simulink model "project3_bonus_2016b"  (R2016b)
settings: Solver=ode23tb  StartTime=0.0  StopTime=inf  MaxStep=1  MinStep=1e-20  RelTol=1e-3
values from neighbouring files (symbols this model uses):
  C1 = 3.5e4    (= 35000)    [init.m]
  Np = 6    [init.m]
  Ns = 100    [init.m]
  Q_cell = Capacity*3600    (= 111600)    [init.m]
  R0 = 0.009    [init.m]
  R1 = 0.0015    [init.m]
  SOC_min = 0.2    [init.m]
undefined symbols (not defined in the file or in its folder): P_trac
libraries: simulink x1
settings Model: Creator=wasynczu  LastModifiedBy=wasynczu
settings SFSimCC: SimUseLocalCustomCode=on
settings RTWCC: RTWUseLocalCustomCode=on

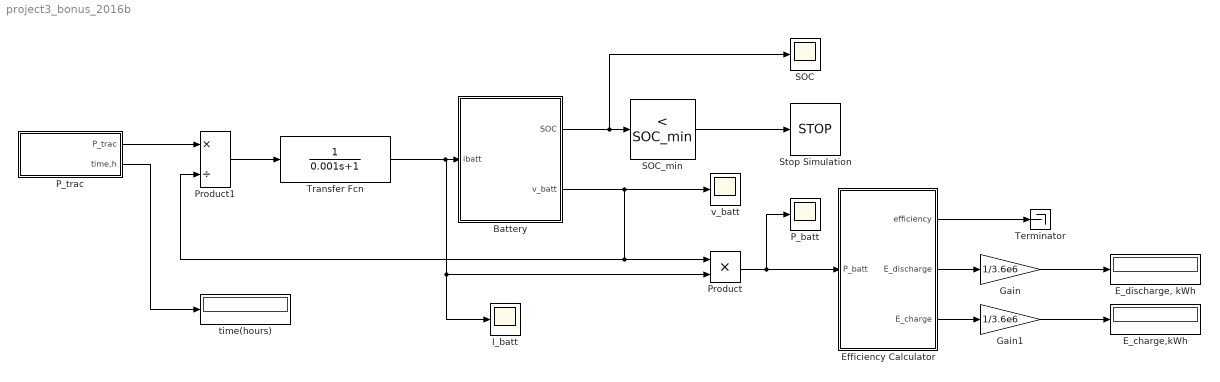
== system project3_bonus_2016b ==
  Battery : Subsystem  mask{SOC_init=1}
      mask prompts: SOC_init "Initial SOC"
  E_charge,kWh : Display
  "E_discharge, kWh" : Display
  Efficiency Calculator : Subsystem
  Gain : Gain  Gain=1/3.6e6
  Gain1 : Gain  Gain=1/3.6e6
  I_batt : Scope
  P_batt : Scope
  P_trac : Subsystem  mask{P_trac=P_trac}
      mask init:
      | N=length(P_trac(1,:))
  Product : Product
  Product1 : Product  Inputs=*/
  SOC : Scope
  SOC_min : simulink/Logic and Bit Operations/Compare To Constant  relop=<  const=SOC_min  OutDataTypeStr=boolean
  Stop Simulation : Stop
  Terminator : Terminator
  Transfer Fcn : TransferFcn  Denominator=[0.001 1]
  time(hours) : Display
  v_batt : Scope
  wires:
  Product1/1 -> Transfer Fcn/1
  Product/1 -> Efficiency Calculator/1(P_batt), P_batt/1
  P_trac/1(P_trac) -> Product1/1
  Battery/2(v_batt) -> Product1/2, Product/1, v_batt/1
  Transfer Fcn/1 -> I_batt/1, Product/2, Battery/1(ibatt)
  SOC_min/1 -> Stop Simulation/1
  Battery/1(SOC) -> SOC/1, SOC_min/1
  Gain1/1 -> E_charge,kWh/1
  Efficiency Calculator/2(E_discharge) -> Gain/1
  Efficiency Calculator/1(efficiency) -> Terminator/1
  Efficiency Calculator/3(E_charge) -> Gain1/1
  Gain/1 -> "E_discharge, kWh"/1
  P_trac/2(time,h) -> time(hours)/1

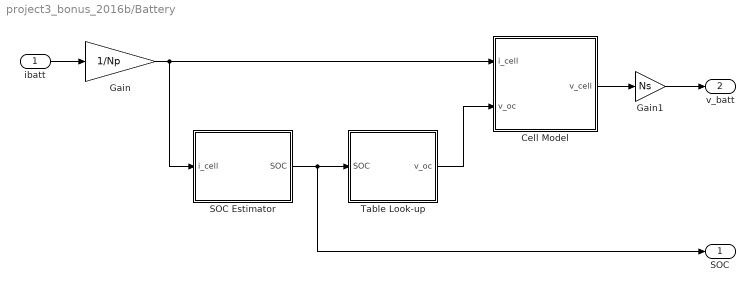
== system project3_bonus_2016b/Battery ==
  ibatt : Inport
  Cell Model : Subsystem  mask{R0=R0, R1=R1, C1=C1, i_cell_init=0}
  Gain : Gain  Gain=1/Np
  Gain1 : Gain  Gain=Ns
  SOC Estimator : Subsystem  mask{SOC_init=SOC_init}
  Table Look-up : Subsystem
  SOC : Outport
  v_batt : Outport  Port=2
  wires:
  Cell Model/1(v_cell) -> Gain1/1
  ibatt/1 -> Gain/1
  Gain1/1 -> v_batt/1
  Table Look-up/1(v_oc) -> Cell Model/2("v_oc ")
  Gain/1 -> SOC Estimator/1(i_cell), Cell Model/1(i_cell)
  SOC Estimator/1(SOC) -> SOC/1, Table Look-up/1(SOC)

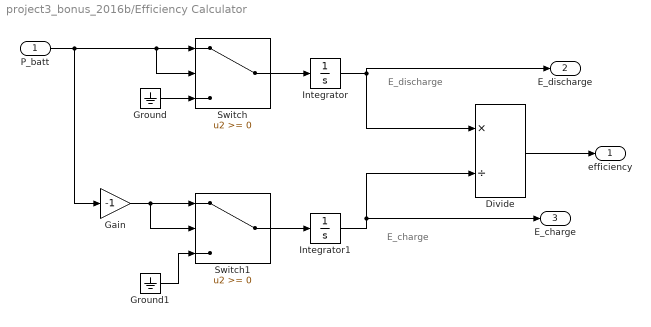
== system project3_bonus_2016b/Efficiency Calculator ==
  note: E_charge
  note: E_discharge
  P_batt : Inport
  Divide : Product  Inputs=*/
  Gain : Gain  Gain=-1
  Ground : Ground
  Ground1 : Ground
  Integrator : Integrator
  Integrator1 : Integrator
  Switch : Switch
  Switch1 : Switch
  efficiency : Outport
  E_discharge : Outport  Port=2
  E_charge : Outport  Port=3
  wires:
  P_batt/1 -> Gain/1, Switch/2, Switch/1
  Ground/1 -> Switch/3
  Gain/1 -> Switch1/2, Switch1/1
  Ground1/1 -> Switch1/3
  Switch/1 -> Integrator/1
  Switch1/1 -> Integrator1/1
  Integrator1/1 -> E_charge/1, Divide/2
  Divide/1 -> efficiency/1
  Integrator/1 -> Divide/1, E_discharge/1

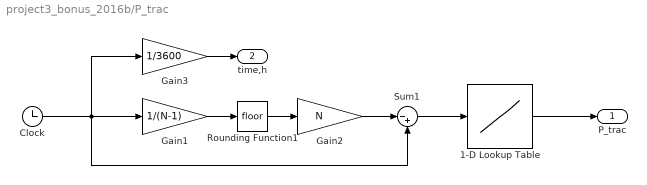
== system project3_bonus_2016b/P_trac ==
  1-D Lookup Table : Lookup_n-D  NumberOfTableDimensions=1  BreakpointsForDimension1=P_trac(1,:)  Table=P_trac(2,:)  InternalRulePriority=Speed  RndMeth=Simplest  InputSameDT=on
  Clock : Clock
  Gain1 : Gain  Gain=1/(N-1)
  Gain2 : Gain  Gain=N
  Gain3 : Gain  Gain=1/3600
  Rounding Function1 : Rounding
  Sum1 : Sum  Inputs=|-+
  P_trac : Outport
  time,h : Outport  Port=2
  wires:
  Clock/1 -> Gain3/1, Gain1/1, Sum1/2
  Sum1/1 -> 1-D Lookup Table/1
  Gain2/1 -> Sum1/1
  Rounding Function1/1 -> Gain2/1
  Gain1/1 -> Rounding Function1/1
  1-D Lookup Table/1 -> P_trac/1
  Gain3/1 -> time,h/1

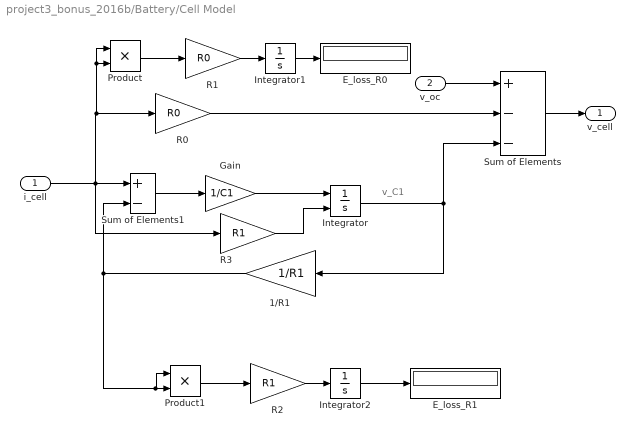
== system project3_bonus_2016b/Battery/Cell Model ==
  note: v_C1
  i_cell : Inport
  "v_oc " : Inport  Port=2
  1/R1 : Gain  Gain=1/R1
  E_loss_R0 : Display
  E_loss_R1 : Display
  Gain : Gain  Gain=1/C1
  Integrator : Integrator  InitialConditionSource=external  InitialCondition=i_cell_init*R1
  Integrator1 : Integrator
  Integrator2 : Integrator
  Product : Product
  Product1 : Product
  R0 : Gain  Gain=R0
  R1 : Gain  Gain=R0
  R2 : Gain  Gain=R1
  R3 : Gain  Gain=R1
  Sum of Elements : Sum  Inputs=+--
  Sum of Elements1 : Sum  Inputs=+-
  v_cell : Outport
  wires:
  "v_oc "/1 -> Sum of Elements/1
  R0/1 -> Sum of Elements/2
  Sum of Elements1/1 -> Gain/1
  Gain/1 -> Integrator/1
  Sum of Elements/1 -> v_cell/1
  Integrator/1 -> Sum of Elements/3, 1/R1/1
  Product/1 -> R1/1
  R1/1 -> Integrator1/1
  Integrator1/1 -> E_loss_R0/1
  R2/1 -> Integrator2/1
  Integrator2/1 -> E_loss_R1/1
  1/R1/1 -> Product1/1, Product1/2, Sum of Elements1/2
  Product1/1 -> R2/1
  R3/1 -> Integrator/2
  i_cell/1 -> R3/1, Product/1, Product/2, R0/1, Sum of Elements1/1

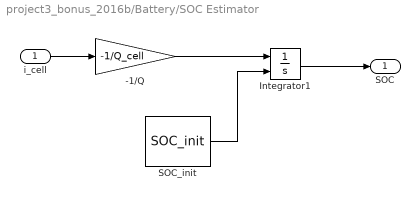
== system project3_bonus_2016b/Battery/SOC Estimator ==
  i_cell : Inport
  -1/Q : Gain  Gain=-1/Q_cell
  Integrator1 : Integrator  InitialConditionSource=external
  SOC_init : Constant  Value=SOC_init
  SOC : Outport
  wires:
  i_cell/1 -> -1/Q/1
  -1/Q/1 -> Integrator1/1
  Integrator1/1 -> SOC/1
  SOC_init/1 -> Integrator1/2

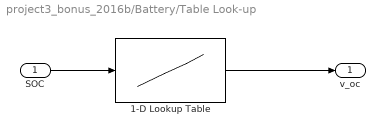
== system project3_bonus_2016b/Battery/Table Look-up ==
  SOC : Inport
  1-D Lookup Table : Lookup_n-D  NumberOfTableDimensions=1  BreakpointsForDimension1=[0 0.1 0.25 0.5 0.75 0.9 1]  Table="[ 3.51  3.57  3.63  3.71  3.93  4.08  4.19]"  RndMeth=Simplest  InputSameDT=on
  v_oc : Outport
  wires:
  SOC/1 -> 1-D Lookup Table/1
  1-D Lookup Table/1 -> v_oc/1
